simulink model "mmodel_dcMotor"  (R2020a)
settings: Solver=ode4  StartTime=0.0  StopTime=15  FixedStep=10e-6  RelTol=1e-3
values from neighbouring files (symbols this model uses):
  flux_nom = En/wn    [mjs.m]
  J = 0.11    [mjs.m]
  kw = (me_nom-mm)/wn^2    [mjs.m]
  La = 30.3e-3    (= 0.0303)    [mjs.m]
  mm_nom = me_nom - kw*wn    [mjs.m]
  Ra = 2.5    [mjs.m]
  Ua = Uan    (= 400)    [mjs.m]
libraries: simulink x1
settings Model: Creator=X  LastModifiedBy=X

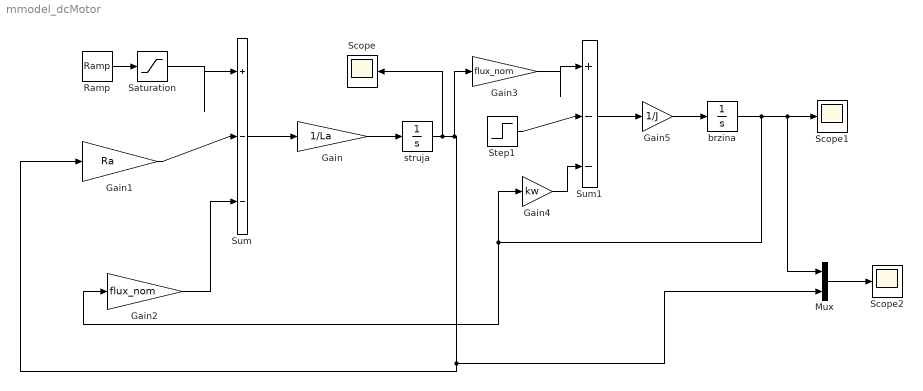
== system mmodel_dcMotor ==
  Gain : Gain  Gain=1/La
  Gain1 : Gain  Gain=Ra
  Gain2 : Gain  Gain=flux_nom
  Gain3 : Gain  Gain=flux_nom
  Gain4 : Gain  Gain=kw
  Gain5 : Gain  Gain=1/J
  Mux : Mux  Inputs=2
  Ramp : simulink/Sources/Ramp  slope=133.33  start=2  InitialOutput=0
  Saturation : Saturate  UpperLimit=Ua  LowerLimit=0
  Scope : Scope
  Scope1 : Scope
  Scope2 : Scope
  Step1 : Step  Time=7  After=mm_nom  SampleTime=0
  Sum : Sum  Inputs=|+--
  Sum1 : Sum  Inputs=|+--
  brzina : Integrator
  struja : Integrator
  wires:
  Gain1/1 -> Sum/2
  Gain2/1 -> Sum/3
  Sum/1 -> Gain/1
  Gain/1 -> struja/1
  Gain3/1 -> Sum1/1
  Gain4/1 -> Sum1/3
  Sum1/1 -> Gain5/1
  Gain5/1 -> brzina/1
  brzina/1 -> Mux/1, Scope1/1, Gain2/1, Gain4/1
  Saturation/1 -> Sum/1
  Ramp/1 -> Saturation/1
  Step1/1 -> Sum1/2
  struja/1 -> Scope/1, Gain3/1, Mux/2, Gain1/1
  Mux/1 -> Scope2/1
